simulink model "MyModel_v0_1"  (R2018b)
settings: Solver=VariableStepAuto  StartTime=0.0  StopTime=10.0  RelTol=1e-3
libraries: powerlib x18, powerlib_meascontrol x4
settings Model: Creator=chenhao  LastModifiedBy=chenhao

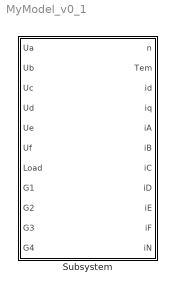
== system MyModel_v0_1 ==
  Subsystem : Subsystem

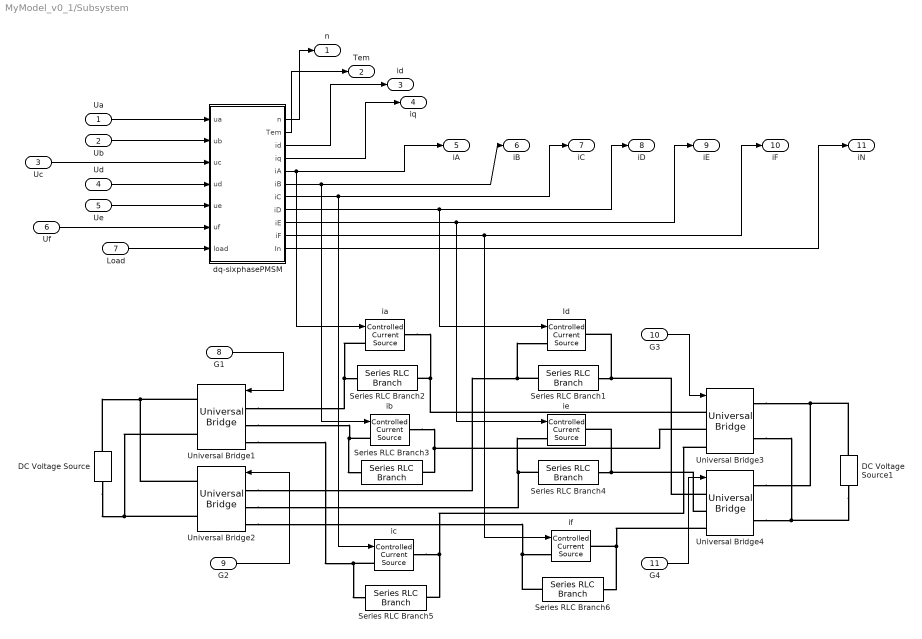
== system MyModel_v0_1/Subsystem ==
  Ua : Inport
  "Ub " : Inport  Port=2
  Uc : Inport  Port=3
  Ud : Inport  Port=4
  Ue : Inport  Port=5
  Uf : Inport  Port=6
  "Load " : Inport  Port=7
  G1 : Inport  Port=8
  G2 : Inport  Port=9
  G3 : Inport  Port=10
  G4 : Inport  Port=11
  DC Voltage Source : powerlib/Electrical Sources/DC Voltage Source  Amplitude=100  Measurements=Voltage
  DC Voltage Source1 : powerlib/Electrical Sources/DC Voltage Source  Amplitude=100  Measurements=Voltage
  Id : powerlib/Electrical Sources/Controlled Current Source  Initialize=on  Source_Type=AC  Amplitude=0  Phase=0  Frequency=0  Measurements=None
  Series RLC Branch{1..6} (6 alike) : powerlib/Elements/Series RLC Branch  LConnTagsString=__new0  RConnTagsString=__new0  BranchType=R  Resistance=10e10  Inductance=10e-7  SetiL0=off  InitialCurrent=0  Capacitance=1e-6  Setx0=off  InitialVoltage=0  Measurements=None
  Universal Bridge{1..4} (4 alike) : powerlib/Power Electronics/Universal Bridge  Arms=3  SnubberResistance=1e5  SnubberCapacitance=inf  Device=IGBT / Diodes  Ron=1e-3  Lon=0  ForwardVoltages="[  0  0  ]"  ForwardVoltage=0  GTOparameters=[ 10e-6 , 20e-6 ]  IGBTparameters=[ 0 , 0 ]  Measurements=None  Measurements_2=None  converterType=Rectifier
  dq-sixphasePMSM : Subsystem  mask{R=0.099, Ld=2.46068e-3, Lq=2.4759e-3, Lf=1.520747e-3, psi=0.0592, p=5, J=0.00174}
      mask prompts: R "Resistance (Om)"; Ld "d-inductance (H)"; Lq "q-inductance (H)"; Lf "Leak inductance (H)"; psi "flux (Wb)"; p "pole pairs"; J "inertia (kg*m^2)"
  ia : powerlib/Electrical Sources/Controlled Current Source  Initialize=on  Source_Type=AC  Amplitude=0  Phase=0  Frequency=0  Measurements=None
  ib : powerlib/Electrical Sources/Controlled Current Source  Initialize=on  Source_Type=AC  Amplitude=0  Phase=0  Frequency=0  Measurements=None
  ic : powerlib/Electrical Sources/Controlled Current Source  Initialize=on  Source_Type=AC  Amplitude=0  Phase=0  Frequency=0  Measurements=None
  ie : powerlib/Electrical Sources/Controlled Current Source  Initialize=on  Source_Type=AC  Amplitude=0  Phase=0  Frequency=0  Measurements=None
  if : powerlib/Electrical Sources/Controlled Current Source  Initialize=on  Source_Type=AC  Amplitude=0  Phase=0  Frequency=0  Measurements=None
  n : Outport
  Tem : Outport  Port=2
  id : Outport  Port=3
  iq : Outport  Port=4
  iA : Outport  Port=5
  iB : Outport  Port=6
  iC : Outport  Port=7
  iD : Outport  Port=8
  iE : Outport  Port=9
  iF : Outport  Port=10
  iN : Outport  Port=11
  wires:
  "Ub "/1 -> dq-sixphasePMSM/2(ub)
  Ua/1 -> dq-sixphasePMSM/1(ua)
  Uc/1 -> dq-sixphasePMSM/3(uc)
  Ud/1 -> dq-sixphasePMSM/4(ud)
  Ue/1 -> dq-sixphasePMSM/5(ue)
  Uf/1 -> dq-sixphasePMSM/6(uf)
  "Load "/1 -> dq-sixphasePMSM/7(load)
  dq-sixphasePMSM/1(n) -> n/1
  dq-sixphasePMSM/2(Tem) -> Tem/1
  dq-sixphasePMSM/3(id) -> id/1
  dq-sixphasePMSM/4(iq) -> iq/1
  dq-sixphasePMSM/5(iA) -> ia/1, iA/1
  dq-sixphasePMSM/6(iB) -> ib/1, iB/1
  dq-sixphasePMSM/7(iC) -> ic/1, iC/1
  dq-sixphasePMSM/8(iD) -> iD/1, Id/1
  dq-sixphasePMSM/9(iE) -> iE/1, ie/1
  dq-sixphasePMSM/10(iF) -> if/1, iF/1
  dq-sixphasePMSM/11(In) -> iN/1
  G1/1 -> Universal Bridge1/1
  G2/1 -> Universal Bridge2/1
  G3/1 -> Universal Bridge3/1
  G4/1 -> Universal Bridge4/1
  connections:
  Series RLC Branch1/RConn1 -- Universal Bridge4/LConn1 -- Id/RConn1
  Series RLC Branch1/LConn1 -- Universal Bridge2/LConn1 -- Id/LConn1
  Series RLC Branch4/RConn1 -- Universal Bridge4/LConn2 -- ie/RConn1
  Series RLC Branch4/LConn1 -- Universal Bridge2/LConn2 -- ie/LConn1
  Series RLC Branch6/LConn1 -- Universal Bridge2/LConn3 -- if/LConn1
  Series RLC Branch6/RConn1 -- Universal Bridge4/LConn3 -- if/RConn1
  Universal Bridge1/RConn2 -- Universal Bridge2/RConn2 -- DC Voltage Source/LConn1
  DC Voltage Source/RConn1 -- Universal Bridge2/RConn1 -- Universal Bridge1/RConn1
  ia/LConn1 -- Universal Bridge1/LConn1 -- Series RLC Branch2/LConn1
  ia/RConn1 -- Universal Bridge3/LConn1 -- Series RLC Branch2/RConn1
  ib/LConn1 -- Universal Bridge1/LConn2 -- Series RLC Branch3/LConn1
  ib/RConn1 -- Universal Bridge3/LConn2 -- Series RLC Branch3/RConn1
  ic/LConn1 -- Series RLC Branch5/LConn1 -- Universal Bridge1/LConn3
  ic/RConn1 -- Universal Bridge3/LConn3 -- Series RLC Branch5/RConn1
  Universal Bridge3/RConn1 -- DC Voltage Source1/RConn1 -- Universal Bridge4/RConn1
  Universal Bridge3/RConn2 -- DC Voltage Source1/LConn1 -- Universal Bridge4/RConn2

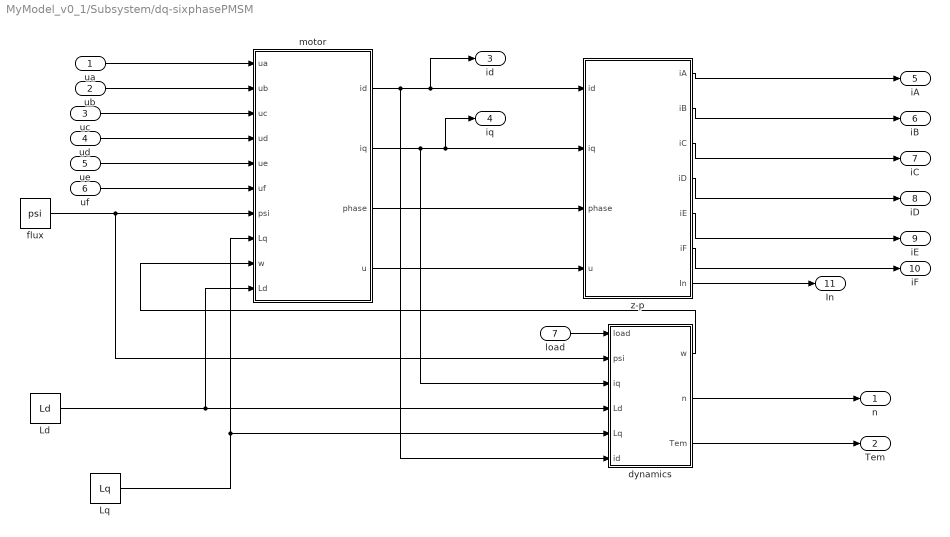
== system MyModel_v0_1/Subsystem/dq-sixphasePMSM ==
  ua : Inport
  ub : Inport  Port=2
  uc : Inport  Port=3
  ud : Inport  Port=4
  ue : Inport  Port=5
  uf : Inport  Port=6
  load : Inport  Port=7
  Ld : Constant  Value=Ld
  Lq : Constant  Value=Lq
  dynamics : Subsystem
  flux : Constant  Value=psi
  motor : Subsystem
  z-p : Subsystem
  n : Outport
  Tem : Outport  Port=2
  id : Outport  Port=3
  iq : Outport  Port=4
  iA : Outport  Port=5
  iB : Outport  Port=6
  iC : Outport  Port=7
  iD : Outport  Port=8
  iE : Outport  Port=9
  iF : Outport  Port=10
  In : Outport  Port=11
  wires:
  Lq/1 -> motor/8(Lq), dynamics/5(Lq)
  Ld/1 -> dynamics/4(Ld), motor/10(Ld)
  ud/1 -> motor/4(ud)
  ua/1 -> motor/1(ua)
  ue/1 -> motor/5(ue)
  ub/1 -> motor/2(ub)
  uf/1 -> motor/6(uf)
  uc/1 -> motor/3(uc)
  dynamics/2(n) -> n/1
  load/1 -> dynamics/1(load)
  z-p/1(iA) -> iA/1
  motor/1(id) -> dynamics/6(id), z-p/1(id), id/1
  motor/2(iq) -> dynamics/3(iq), z-p/2(iq), iq/1
  motor/4(u) -> z-p/4(u)
  dynamics/1(w) -> motor/9(w)
  dynamics/3(Tem) -> Tem/1
  flux/1 -> dynamics/2(psi), motor/7(psi)
  z-p/2(iB) -> iB/1
  z-p/3(iC) -> iC/1
  z-p/4(iD) -> iD/1
  z-p/5(iE) -> iE/1
  z-p/6(iF) -> iF/1
  motor/3(phase) -> z-p/3(phase)
  z-p/7(In) -> In/1

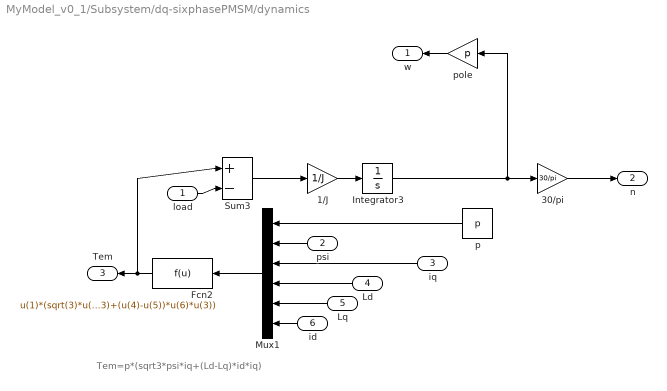
== system MyModel_v0_1/Subsystem/dq-sixphasePMSM/dynamics ==
  note: Tem=p*(sqrt3*psi*iq+(Ld-Lq)*id*iq)
  load : Inport
  psi : Inport  Port=2
  iq : Inport  Port=3
  Ld : Inport  Port=4
  Lq : Inport  Port=5
  id : Inport  Port=6
  1/J : Gain  Gain=1/J  SaturateOnIntegerOverflow=on  OutDataTypeStr=Inherit: Same as input  ParamDataTypeStr=Inherit: Same as input
  30/pi : Gain  Gain=30/pi  SaturateOnIntegerOverflow=on  OutDataTypeStr=Inherit: Same as input  ParamDataTypeStr=Inherit: Same as input
  Fcn2 : Fcn  Expr=u(1)*(sqrt(3)*u(2)*u(3)+(u(4)-u(5))*u(6)*u(3))
  Integrator3 : Integrator
  Mux1 : Mux  Inputs=6
  Sum3 : Sum  Inputs=|+-  SaturateOnIntegerOverflow=on
  p : Constant  Value=p
  pole : Gain  Gain=p  SaturateOnIntegerOverflow=on  OutDataTypeStr=Inherit: Same as input  ParamDataTypeStr=Inherit: Same as input
  w : Outport
  n : Outport  Port=2
  Tem : Outport  Port=3
  wires:
  p/1 -> Mux1/1
  Mux1/1 -> Fcn2/1
  Fcn2/1 -> Sum3/1, Tem/1
  Sum3/1 -> 1/J/1
  1/J/1 -> Integrator3/1
  Integrator3/1 -> 30/pi/1, pole/1
  psi/1 -> Mux1/2
  Ld/1 -> Mux1/4
  Lq/1 -> Mux1/5
  pole/1 -> w/1
  30/pi/1 -> n/1
  load/1 -> Sum3/2
  iq/1 -> Mux1/3
  id/1 -> Mux1/6

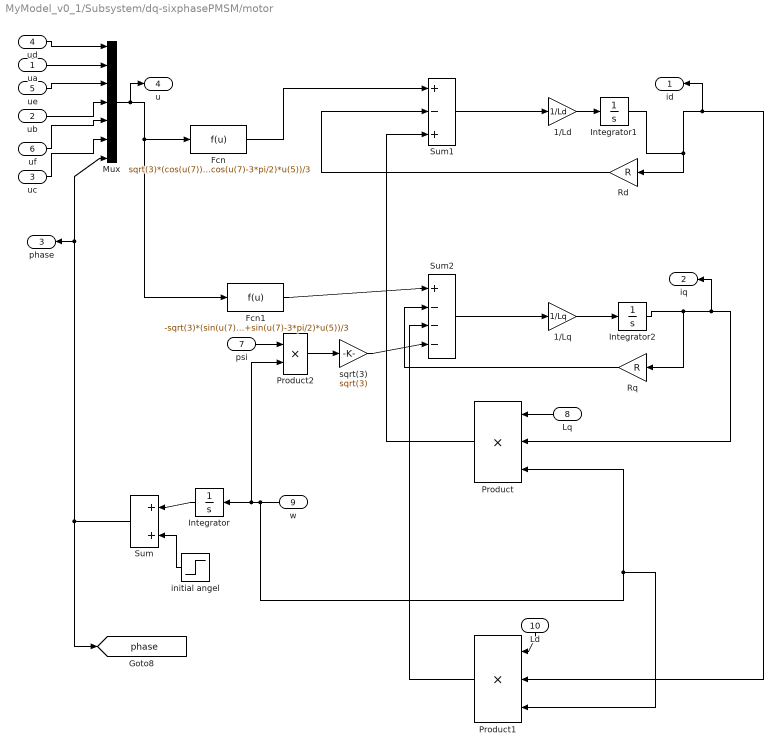
== system MyModel_v0_1/Subsystem/dq-sixphasePMSM/motor ==
  ua : Inport
  ub : Inport  Port=2
  uc : Inport  Port=3
  ud : Inport  Port=4
  ue : Inport  Port=5
  uf : Inport  Port=6
  psi : Inport  Port=7
  Lq : Inport  Port=8
  w : Inport  Port=9
  Ld : Inport  Port=10
  1/Ld : Gain  Gain=1/Ld  SaturateOnIntegerOverflow=on  OutDataTypeStr=Inherit: Same as input  ParamDataTypeStr=Inherit: Same as input
  1/Lq : Gain  Gain=1/Lq  SaturateOnIntegerOverflow=on  OutDataTypeStr=Inherit: Same as input  ParamDataTypeStr=Inherit: Same as input
  Fcn : Fcn  Expr=sqrt(3)*(cos(u(7))*u(2)+cos(u(7)-pi/6)*u(4)+cos(u(7)-2*pi/3)*u(6)+cos(u(7)-5*pi/6)*u(1)+cos(u(7)-4*pi/3)*u(3)+cos(u(7)-3*pi/2)*u(5))/3
  Fcn1 : Fcn  Expr=-sqrt(3)*(sin(u(7))*u(2)+sin(u(7)-pi/6)*u(4)+sin(u(7)-2*pi/3)*u(6)+sin(u(7)-5*pi/6)*u(1)+sin(u(7)-4*pi/3)*u(3)+sin(u(7)-3*pi/2)*u(5))/3
  Integrator : Integrator
  Integrator1 : Integrator
  Integrator2 : Integrator
  Mux : Mux  Inputs=7
  Product : Product  Inputs=3  SaturateOnIntegerOverflow=on  OutDataTypeStr=Inherit: Same as first input
  Product1 : Product  Inputs=3  SaturateOnIntegerOverflow=on  OutDataTypeStr=Inherit: Same as first input
  Product2 : Product  SaturateOnIntegerOverflow=on  OutDataTypeStr=Inherit: Same as first input
  Rd : Gain  Gain=R  SaturateOnIntegerOverflow=on  OutDataTypeStr=Inherit: Same as input  ParamDataTypeStr=Inherit: Same as input
  Rq : Gain  Gain=R  SaturateOnIntegerOverflow=on  OutDataTypeStr=Inherit: Same as input  ParamDataTypeStr=Inherit: Same as input
  Sum : Sum  Inputs=|++  SaturateOnIntegerOverflow=on
  Sum1 : Sum  Inputs=|+-+  SaturateOnIntegerOverflow=on
  Sum2 : Sum  Inputs=|+---  SaturateOnIntegerOverflow=on
  initial angel : Step  Time=0  After=13*pi/9  SampleTime=0
  sqrt(3) : Gain  Gain=sqrt(3)  SaturateOnIntegerOverflow=on  OutDataTypeStr=Inherit: Same as input  ParamDataTypeStr=Inherit: Same as input
  id : Outport
  iq : Outport  Port=2
  phase : Outport  Port=3
  u : Outport  Port=4
  tag scope: phase=global
  wires:
  Sum/1 -> Mux/7, phase/1, [phase]
  Integrator/1 -> Sum/1
  initial angel/1 -> Sum/2
  w/1 -> Product2/2, Integrator/1, Product1/3, Product/3
  Mux/1 -> Fcn/1, Fcn1/1, u/1
  Fcn/1 -> Sum1/1
  Sum1/1 -> 1/Ld/1
  1/Ld/1 -> Integrator1/1
  Integrator1/1 -> Rd/1, id/1, Product1/2
  Rd/1 -> Sum1/2
  Fcn1/1 -> Sum2/1
  Sum2/1 -> 1/Lq/1
  1/Lq/1 -> Integrator2/1
  Integrator2/1 -> Rq/1, iq/1, Product/2
  Rq/1 -> Sum2/2
  Product/1 -> Sum1/3
  Product1/1 -> Sum2/3
  Product2/1 -> sqrt(3)/1
  psi/1 -> Product2/1
  Lq/1 -> Product/1
  Ld/1 -> Product1/1
  ud/1 -> Mux/1
  ua/1 -> Mux/2
  ue/1 -> Mux/3
  ub/1 -> Mux/4
  uf/1 -> Mux/5
  uc/1 -> Mux/6
  sqrt(3)/1 -> Sum2/4

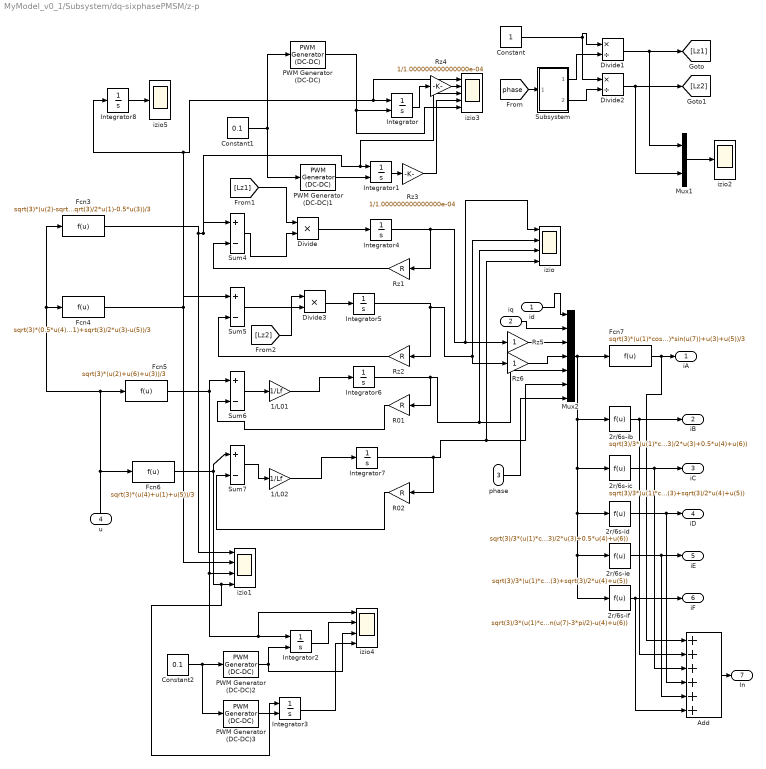
== system MyModel_v0_1/Subsystem/dq-sixphasePMSM/z-p ==
  id : Inport
  iq : Inport  Port=2
  phase : Inport  Port=3
  u : Inport  Port=4
  1/L01 : Gain  Gain=1/Lf  SaturateOnIntegerOverflow=on  OutDataTypeStr=Inherit: Same as input  ParamDataTypeStr=Inherit: Same as input
  1/L02 : Gain  Gain=1/Lf  SaturateOnIntegerOverflow=on  OutDataTypeStr=Inherit: Same as input  ParamDataTypeStr=Inherit: Same as input
  2r/6s-ib : Fcn  Expr=sqrt(3)/3*(u(1)*cos(u(7)-pi/6)-u(2)*sin(u(7)-pi/6)-sqrt(3)/2*u(3)+0.5*u(4)+u(6))
  2r/6s-ic : Fcn  Expr=sqrt(3)/3*(u(1)*cos(u(7)-2*pi/3)-u(2)*sin(u(7)-2*pi/3)-0.5*u(3)+sqrt(3)/2*u(4)+u(5))
  2r/6s-id : Fcn  Expr=sqrt(3)/3*(u(1)*cos(u(7)-5*pi/6)-u(2)*sin(u(7)-5*pi/6)+sqrt(3)/2*u(3)+0.5*u(4)+u(6))
  2r/6s-ie : Fcn  Expr=sqrt(3)/3*(u(1)*cos(u(7)-4*pi/3)-u(2)*sin(u(7)-4*pi/3)-0.5*u(3)+sqrt(3)/2*u(4)+u(5))
  2r/6s-if : Fcn  Expr=sqrt(3)/3*(u(1)*cos(u(7)-3*pi/2)-u(2)*sin(u(7)-3*pi/2)-u(4)+u(6))
  Add : Sum  Inputs=++++++
  Constant : Constant
  Constant1 : Constant  Value=0.1
  Constant2 : Constant  Value=0.1
  Divide : Product  Inputs=**
  Divide1 : Product  Inputs=*/
  Divide2 : Product  Inputs=*/
  Divide3 : Product  Inputs=**
  Fcn3 : Fcn  Expr=sqrt(3)*(u(2)-sqrt(3)/2*u(4)-0.5*u(6)+sqrt(3)/2*u(1)-0.5*u(3))/3
  Fcn4 : Fcn  Expr=sqrt(3)*(0.5*u(4)-sqrt(3)/2*u(6)+0.5*u(1)+sqrt(3)/2*u(3)-u(5))/3
  Fcn5 : Fcn  Expr=sqrt(3)*(u(2)+u(6)+u(3))/3
  Fcn6 : Fcn  Expr=sqrt(3)*(u(4)+u(1)+u(5))/3
  Fcn7 : Fcn  Expr=sqrt(3)*(u(1)*cos(u(7))-u(2)*sin(u(7))+u(3)+u(5))/3
  Integrator{,1..3} (4 alike) : Integrator  ExternalReset=rising
  Integrator{4..8} (5 alike) : Integrator
  Mux1 : Mux  Inputs=2
  Mux2 : Mux  Inputs=7
  PWM Generator (DC-DC){,1..3} (4 alike) : powerlib_meascontrol/Pulse & Signal Generators/PWM Generator (DC-DC)  Fsw=1/1.000000000000000e-04  Ts=0
  R01 : Gain  Gain=R  SaturateOnIntegerOverflow=on  OutDataTypeStr=Inherit: Same as input  ParamDataTypeStr=Inherit: Same as input
  R02 : Gain  Gain=R  SaturateOnIntegerOverflow=on  OutDataTypeStr=Inherit: Same as input  ParamDataTypeStr=Inherit: Same as input
  Rz1 : Gain  Gain=R  SaturateOnIntegerOverflow=on  OutDataTypeStr=Inherit: Same as input  ParamDataTypeStr=Inherit: Same as input
  Rz2 : Gain  Gain=R  SaturateOnIntegerOverflow=on  OutDataTypeStr=Inherit: Same as input  ParamDataTypeStr=Inherit: Same as input
  Rz3 : Gain  Gain=1/1.000000000000000e-04  SaturateOnIntegerOverflow=on  OutDataTypeStr=Inherit: Same as input  ParamDataTypeStr=Inherit: Same as input
  Rz4 : Gain  Gain=1/1.000000000000000e-04  SaturateOnIntegerOverflow=on  OutDataTypeStr=Inherit: Same as input  ParamDataTypeStr=Inherit: Same as input
  Rz5 : Gain  SaturateOnIntegerOverflow=on  OutDataTypeStr=Inherit: Same as input  ParamDataTypeStr=Inherit: Same as input
  Rz6 : Gain  SaturateOnIntegerOverflow=on  OutDataTypeStr=Inherit: Same as input  ParamDataTypeStr=Inherit: Same as input
  Subsystem : Subsystem
  Sum{4..7} (4 alike) : Sum  Inputs=|+-  SaturateOnIntegerOverflow=on
  izio : Scope  NumInputPorts=4
  izio1 : Scope  NumInputPorts=4
  izio2 : Scope
  izio3 : Scope  NumInputPorts=5
  izio4 : Scope  NumInputPorts=4
  izio5 : Scope
  iA : Outport
  iB : Outport  Port=2
  iC : Outport  Port=3
  iD : Outport  Port=4
  iE : Outport  Port=5
  iF : Outport  Port=6
  In : Outport  Port=7
  wires:
  Mux2/1 -> Fcn7/1, 2r/6s-ic/1, 2r/6s-id/1, 2r/6s-ie/1, 2r/6s-if/1, 2r/6s-ib/1
  R02/1 -> Sum7/2
  R01/1 -> Sum6/2
  Rz2/1 -> Sum5/2
  Rz1/1 -> Sum4/2
  Integrator7/1 -> R02/1, Mux2/6, izio/4
  1/L02/1 -> Integrator7/1
  Sum7/1 -> 1/L02/1
  Integrator6/1 -> R01/1, Mux2/5, izio/3
  1/L01/1 -> Integrator6/1
  Sum6/1 -> 1/L01/1
  id/1 -> Mux2/1
  iq/1 -> Mux2/2
  u/1 -> Fcn4/1, Fcn3/1, Fcn5/1, Fcn6/1
  phase/1 -> Mux2/7
  Fcn7/1 -> Add/1, iA/1
  2r/6s-ib/1 -> Add/2, iB/1
  2r/6s-id/1 -> Add/4, iD/1
  2r/6s-ie/1 -> Add/5, iE/1
  2r/6s-if/1 -> Add/6, iF/1
  [phase] -> Subsystem/1(Phase)
  Subsystem/1(Lz1) -> Divide1/2
  Divide1/1 -> Mux1/1, [Lz1]
  Constant/1 -> Divide1/1, Divide2/1
  Subsystem/2(Lz2) -> Divide2/2
  Divide2/1 -> Mux1/2, [Lz2]
  Mux1/1 -> izio2/1
  Sum4/1 -> Divide/2
  [Lz1] -> Divide/1
  Divide/1 -> Integrator4/1
  Divide3/1 -> Integrator5/1
  Sum5/1 -> Divide3/2
  [Lz2] -> Divide3/1
  Constant1/1 -> PWM Generator (DC-DC)/1, PWM Generator (DC-DC)1/1
  PWM Generator (DC-DC)/1 -> izio3/5, Integrator/2
  PWM Generator (DC-DC)1/1 -> Integrator1/2
  Fcn6/1 -> Sum7/1, Integrator3/1, izio1/4
  Fcn5/1 -> Sum6/1, izio4/1, Integrator2/1, izio1/3
  Constant2/1 -> PWM Generator (DC-DC)3/1, PWM Generator (DC-DC)2/1
  PWM Generator (DC-DC)2/1 -> Integrator2/2, izio4/3
  Integrator2/1 -> izio4/2
  PWM Generator (DC-DC)3/1 -> Integrator3/2
  Integrator3/1 -> izio4/4
  Integrator1/1 -> Rz3/1
  Rz3/1 -> izio3/4
  Integrator5/1 -> Rz2/1, Rz6/1, izio/2
  Rz4/1 -> izio3/2
  Integrator/1 -> Rz4/1
  Integrator4/1 -> Rz1/1, Rz5/1, izio/1
  Rz5/1 -> Mux2/3
  Rz6/1 -> Mux2/4
  Integrator8/1 -> izio5/1
  Fcn3/1 -> izio1/1, izio3/3, Integrator1/1, Sum4/1
  Fcn4/1 -> Sum5/1, izio3/1, Integrator/1, Integrator8/1, izio1/2
  Add/1 -> In/1
  2r/6s-ic/1 -> Add/3, iC/1

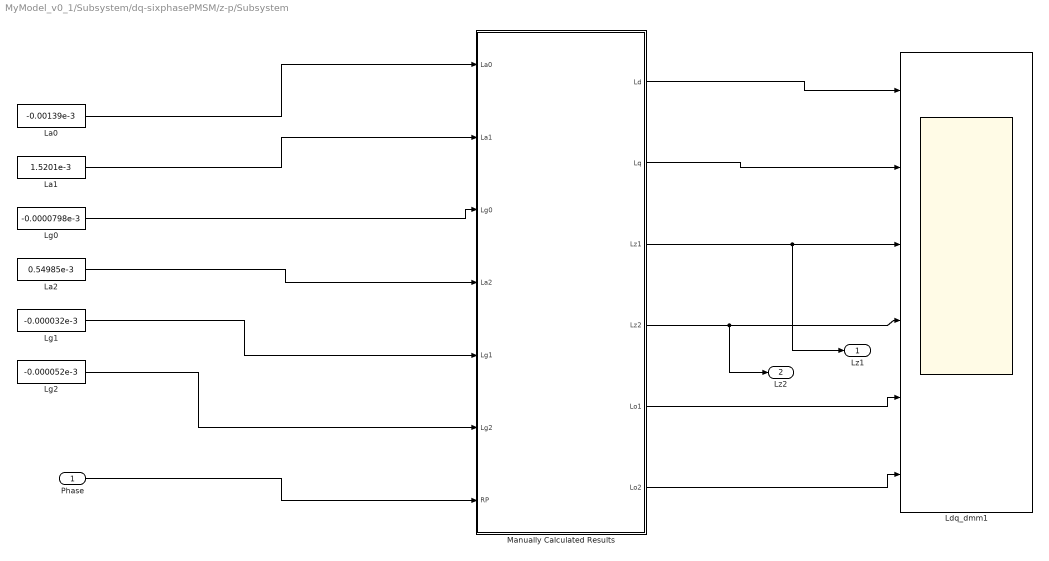
== system MyModel_v0_1/Subsystem/dq-sixphasePMSM/z-p/Subsystem ==
  Phase : Inport
  La0 : Constant  Value=-0.00139e-3
  La1 : Constant  Value=1.5201e-3
  La2 : Constant  Value=0.54985e-3
  Ldq_dmm1 : Scope  NumInputPorts=6
  Lg0 : Constant  Value=-0.0000798e-3
  Lg1 : Constant  Value=-0.000032e-3
  Lg2 : Constant  Value=-0.000052e-3
  "Manually Calculated Results " : MATLAB Function  TreatAsAtomicUnit=on
  Lz1 : Outport
  Lz2 : Outport  Port=2
  wires:
  "Manually Calculated Results "/3(Lz1) -> Lz1/1, Ldq_dmm1/3
  Lg2/1 -> "Manually Calculated Results "/6(Lg2)
  Lg1/1 -> "Manually Calculated Results "/5(Lg1)
  "Manually Calculated Results "/2(Lq) -> Ldq_dmm1/2
  Lg0/1 -> "Manually Calculated Results "/3(Lg0)
  "Manually Calculated Results "/4(Lz2) -> Lz2/1, Ldq_dmm1/4
  "Manually Calculated Results "/6(Lo2) -> Ldq_dmm1/6
  "Manually Calculated Results "/1(Ld) -> Ldq_dmm1/1
  "Manually Calculated Results "/5(Lo1) -> Ldq_dmm1/5
  La0/1 -> "Manually Calculated Results "/1(La0)
  La1/1 -> "Manually Calculated Results "/2(La1)
  La2/1 -> "Manually Calculated Results "/4(La2)
  Phase/1 -> "Manually Calculated Results "/7(RP)

== matlab function MyModel_v0_1/Subsystem/dq-sixphasePMSM/z-p/Subsystem/Manually Calculated Results  ==
  data: La0 input; Ld output; La1 input; Lg0 input; La2 input; Lg1 input; Lg2 input; RP input; Lq output; Lz1 output; Lz2 output; Lo1 output; Lo2 output
function [Ld,Lq,Lz1,Lz2,Lo1,Lo2] = fcn(La0,La1,Lg0,La2,Lg1,Lg2,RP)
%#codegen
Ld=3*La0+La1+sqrt(3)*La2+(1/2*Lg0+Lg1+Lg2);
Lq=3*La0+sqrt(3)*La2+La1-(1/2*Lg0+Lg1+Lg2);
Lz1=La1+cos(2*RP)*(1/2*Lg0-Lg1+Lg2)-sqrt(3)*La2;
Lz2=La1-cos(2*RP)*(1/2*Lg0-Lg1+Lg2)-sqrt(3)*La2;
Lo1=La1;
Lo2=La1;
